simulink model "kelvinVoigtTether_th"  (R2018b)
settings: Solver=ode15s  StartTime=0.0  StopTime=sim_time  MaxStep=dt  RelTol=1e-3
undefined symbols (not defined in the file or in its folder): amp, class_thr, omega
libraries: kelvinVoigtTether_cl x1
settings Model: Creator=Ayaz  LastModifiedBy=Ayaz

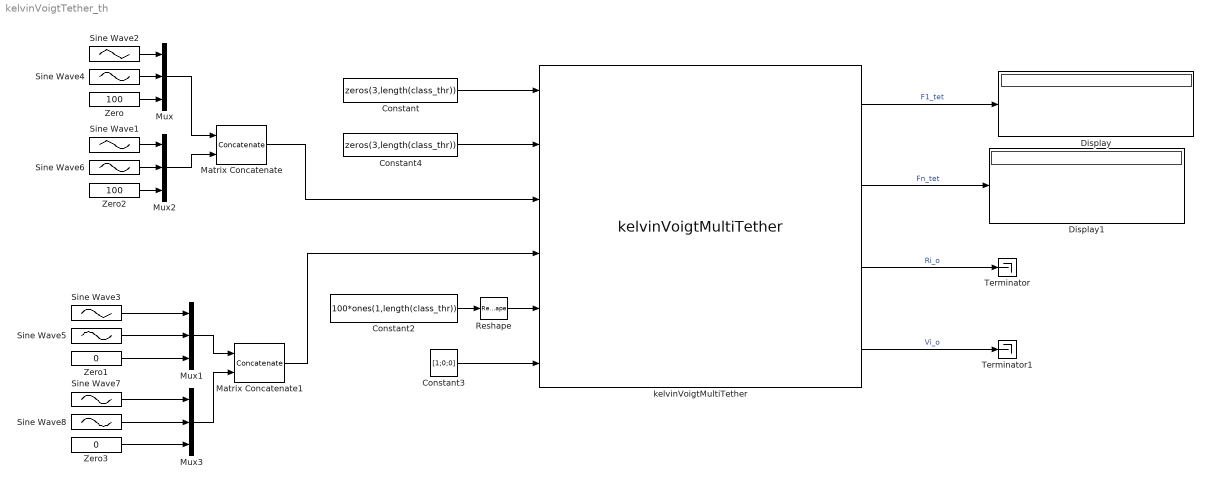
== system kelvinVoigtTether_th ==
  Constant : Constant  Value=zeros(3,length(class_thr))  VectorParams1D=off
  Constant2 : Constant  Value=100*ones(1,length(class_thr))  VectorParams1D=off
  Constant3 : Constant  Value=[1;0;0]  VectorParams1D=off
  Constant4 : Constant  Value=zeros(3,length(class_thr))  VectorParams1D=off
  Display : Display
  Display1 : Display
  Matrix Concatenate : Concatenate  Mode=Multidimensional array  ConcatenateDimension=2
  Matrix Concatenate1 : Concatenate  Mode=Multidimensional array  ConcatenateDimension=2
  Mux{,1..3} (4 alike) : Mux  Inputs=3
  Reshape : Reshape  OutputDimensionality=Row vector (2-D)
  Sine Wave1 : Sin  Amplitude=amp  Frequency=omega  Phase=pi/2  SampleTime=0
  Sine Wave2 : Sin  Amplitude=amp  Frequency=omega  Phase=pi/2  SampleTime=0
  Sine Wave3 : Sin  Amplitude=-amp*omega  Frequency=omega  SampleTime=0
  Sine Wave4 : Sin  Amplitude=amp  Bias=-1  Frequency=omega  SampleTime=0
  Sine Wave5 : Sin  Amplitude=amp*omega  Frequency=omega  Phase=pi/2  SampleTime=0
  Sine Wave6 : Sin  Amplitude=amp  Bias=1  Frequency=omega  SampleTime=0
  Sine Wave7 : Sin  Amplitude=-amp*omega  Frequency=omega  SampleTime=0
  Sine Wave8 : Sin  Amplitude=amp*omega  Frequency=omega  Phase=pi/2  SampleTime=0
  Terminator : Terminator
  Terminator1 : Terminator
  Zero : Constant  Value=100  OutDataTypeStr=Inherit: Inherit via back propagation
  Zero1 : Constant  Value=0  OutDataTypeStr=Inherit: Inherit via back propagation
  Zero2 : Constant  Value=100  OutDataTypeStr=Inherit: Inherit via back propagation
  Zero3 : Constant  Value=0  OutDataTypeStr=Inherit: Inherit via back propagation
  kelvinVoigtMultiTether : kelvinVoigtTether_cl/kelvinVoigtMultiTether  rho_fluid=rho_f  grav=G  M=mass  tN=[class_thr.numNodes]  tD=[class_thr.diameter]  tRho=[class_thr.density]  tE=[class_thr.youngsModulus]  tZeta=[class_thr.dampingRatio]  tCd=[class_thr.dragCoeff]  iniR1_o=[class_thr.ini_R1_o]  iniRn_o=[class_thr.ini_Rn_o]  iniRi_o=n_ini_pos  iniVi_o=n_ini_vel
      link override kelvinVoigtTether: LabelModeActiveChoice=tetherNumNodeN_variant
  wires:
  kelvinVoigtMultiTether/3 -> Terminator/1  "Ri_o"
  kelvinVoigtMultiTether/1 -> Display/1  "F1_tet"
  kelvinVoigtMultiTether/2 -> Display1/1  "Fn_tet"
  kelvinVoigtMultiTether/4 -> Terminator1/1  "Vi_o"
  Constant/1 -> kelvinVoigtMultiTether/1
  Constant4/1 -> kelvinVoigtMultiTether/2
  Constant2/1 -> Reshape/1
  Constant3/1 -> kelvinVoigtMultiTether/6
  Sine Wave4/1 -> Mux/2
  Sine Wave3/1 -> Mux1/1
  Sine Wave2/1 -> Mux/1
  Zero/1 -> Mux/3
  Sine Wave5/1 -> Mux1/2
  Zero1/1 -> Mux1/3
  Zero2/1 -> Mux2/3
  Sine Wave1/1 -> Mux2/1
  Sine Wave6/1 -> Mux2/2
  Mux/1 -> Matrix Concatenate/1
  Mux2/1 -> Matrix Concatenate/2
  Matrix Concatenate/1 -> kelvinVoigtMultiTether/3
  Zero3/1 -> Mux3/3
  Sine Wave8/1 -> Mux3/2
  Sine Wave7/1 -> Mux3/1
  Mux1/1 -> Matrix Concatenate1/1
  Mux3/1 -> Matrix Concatenate1/2
  Matrix Concatenate1/1 -> kelvinVoigtMultiTether/4
  Reshape/1 -> kelvinVoigtMultiTether/5
